simulink model "Tiltrotor_temp"  (R2017b)
settings: Solver=VariableStepAuto  StartTime=0.0  StopTime=60  RelTol=1e-3
PreLoadFcn:
  | parameter_Tiltrotor;
  | time;
InitFcn:
  | parameter_Tiltrotor;
  | time;
model workspace: external: MATLAB File E:\Matlab\CTRUAV_V1\parameter_Tiltrotor.m (data not in the file)
values from neighbouring files (symbols this model uses):
  Bm = 2    [parameter_Tiltrotor.m]
  Dm = 0.005    [parameter_Tiltrotor.m]
  Dphi = 0.01    [parameter_Tiltrotor.m]
  Dpsi = 0.01    [parameter_Tiltrotor.m]
  Ds = 15    [parameter_Tiltrotor.m]
  Dtheta = 0.01    [parameter_Tiltrotor.m]
  Dx = 0.04    [parameter_Tiltrotor.m]
  Dy = 0.04    [parameter_Tiltrotor.m]
  Dz = 0.08    [parameter_Tiltrotor.m]
  Im = 0.05    [parameter_Tiltrotor.m]
  Inheight = 0.1    [parameter_Tiltrotor.m]
  Is = 0    [parameter_Tiltrotor.m]
  Kdphi = 7    [parameter_Tiltrotor.m]
  Kdpsi = 4    [parameter_Tiltrotor.m]
  Kdtheta = 9    [parameter_Tiltrotor.m]
  Kdx = 5    [parameter_Tiltrotor.m]
  Kdy = 3    [parameter_Tiltrotor.m]
  Kdz = 6.5    [parameter_Tiltrotor.m]
  Kf = 0.04    [parameter_Tiltrotor.m]
  Kfv = 0.04    [parameter_Tiltrotor.m]
  Kphi = 7    [parameter_Tiltrotor.m]
  Kpsi = 4    [parameter_Tiltrotor.m]
  Ktheta = 9    [parameter_Tiltrotor.m]
  lb = 0.24    [parameter_Tiltrotor.m]
  lf = 0.078    [parameter_Tiltrotor.m]
  lh = 0.0142    [parameter_Tiltrotor.m]
  ls = 0.151    [parameter_Tiltrotor.m]
  m = 0.979    [parameter_Tiltrotor.m]
  Pm = 0.16    [parameter_Tiltrotor.m]
  Ps = 30    [parameter_Tiltrotor.m]
undefined symbols (not defined in the file or in its folder): sigbuilder_block, smiData, X, Y, Z
libraries: sm_lib x243, nesl_utility x48, simulink x8, fl_lib x4
(part 1 of 6)
settings Model: Creator=Lvzongyang  LastModifiedBy=lvzongyang

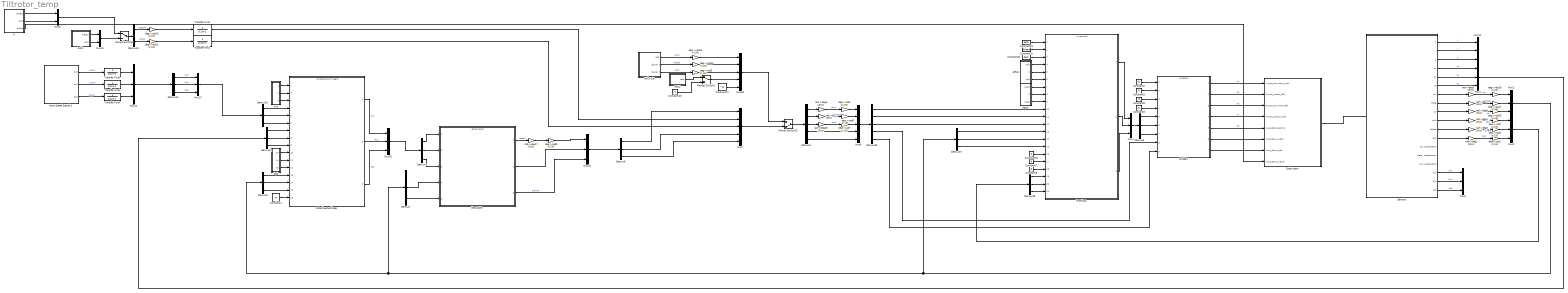
== system Tiltrotor_temp ==
  0 : Subsystem  Tag=STV Subsys  LoadFcn=sigbuilder_block('load');  StartFcn=sigbuilder_block('start');  StopFcn=sigbuilder_block('stop');  ClipboardFcn=sigbuilder_block('clipboard');  mask(Sigbuilder block){tuvar=[0:10]}
      mask help: Simulink:masks:SigbuilderBlock_MD
      mask init:
      | if ~strcmp(get_param(bdroot(gcbh),'SimulationStatus'),'stopped') tuvar = sigbuilder_block('maskInit'); end
      settings: CopyFcn=sigbuilder_block('copy');  DeleteFcn=sigbuilder_block('delete');  ModelCloseFcn=sigbuilder_block('modelClose');  PreSaveFcn=sigbuilder_block('preSave');  PauseFcn=sigbuilder_block('pause');  ContinueFcn=sigbuilder_block('continue');  NameChangeFcn=sigbuilder_block('namechange');  OpenFcn=sigbuilder_block('open',[1322.25 66 1162.5 420.75 ]);  CloseFcn=sigbuilder_block('close');
      mask Display: plot(0, 0, 100, 100,[2, 2, 32, 32, 2], [68, 8, 8, 68, 68],[32, 2], [38, 38], [32, 19, 2],[53, 60, 44], [32, 17, 17, 2],[16, 16, 31, 31]);txt = getActiveGroup(gcbh);text(2, 100, txt,'verticalAlignment', 'top');
  Constant1 : Constant  Value=m
  Constant{7,9..10,15} (4 alike) : Constant  Value=0
  Constant17 : Constant  Value=-11
  Constant19 : Constant  Value=Dphi
  Constant2 : Constant  Value=lb
  Constant20 : Constant  Value=Dtheta
  Constant21 : Constant  Value=Dpsi
  Constant3 : Constant  Value=lf
  Constant6 : Constant  Value=ls
  Constant8 : Constant  Value=lh
  Decoupler : ModelReference  ModelNameDialog=Decoupler0  ModelReferenceVersion=1.160  CopyOfModelProtected=on
  Demux10 : Demux  Outputs=2
  Demux{2..3,7..9,14,20..21,37,39} (10 alike) : Demux  Outputs=3
  Demux36 : Demux  Outputs=5
  Demux6 : Demux  Outputs=5
  Dp2 : Subsystem
  Input Speed Signals1 : Subsystem  Tag=STV Subsys  LoadFcn=sigbuilder_block('load');  StartFcn=sigbuilder_block('start');  StopFcn=sigbuilder_block('stop');  ClipboardFcn=sigbuilder_block('clipboard');  mask(Sigbuilder block){tuvar=[0:10]}
      mask help: Simulink:masks:SigbuilderBlock_MD
      mask init:
      | if ~strcmp(get_param(bdroot(gcbh),'SimulationStatus'),'stopped') tuvar = sigbuilder_block('maskInit'); end
      settings: CopyFcn=sigbuilder_block('copy');  DeleteFcn=sigbuilder_block('delete');  ModelCloseFcn=sigbuilder_block('modelClose');  PreSaveFcn=sigbuilder_block('preSave');  PauseFcn=sigbuilder_block('pause');  ContinueFcn=sigbuilder_block('continue');  NameChangeFcn=sigbuilder_block('namechange');  OpenFcn=sigbuilder_block('open',[57.75 0 966.75 517.5 ]);  CloseFcn=sigbuilder_block('close');
      mask Display: plot(0, 0, 100, 100,[2, 2, 32, 32, 2], [68, 8, 8, 68, 68],[32, 2], [38, 38], [32, 19, 2],[53, 60, 44], [32, 17, 17, 2],[16, 16, 31, 31]);txt = getActiveGroup(gcbh);text(2, 100, txt,'verticalAlignment', 'top');
  Kot : Subsystem
  MIXER1 : ModelReference  ModelNameDialog=MIXER10  ModelReferenceVersion=1.160  CopyOfModelProtected=on
  Manual Switch2 : ManualSwitch
  Manual Switch23 : ManualSwitch  CurrentSetting=0
  Manual Switch6 : ManualSwitch
  Mux{1..5,11..12,19,25,27} (10 alike) : Mux  Inputs=3
  Mux10 : Mux  Inputs=2
  Mux39 : Mux  Inputs=5
  Mux6 : Mux  Inputs=5
  Mux7 : Mux  Inputs=5
  Mux9 : Mux  Inputs=2
  "Outerloopnonlinear " : ModelReference  ModelNameDialog=Outerloopnonlinear0  ModelReferenceVersion=1.160  CopyOfModelProtected=on
  Roll1 : Subsystem  Tag=STV Subsys  LoadFcn=sigbuilder_block('load');  StartFcn=sigbuilder_block('start');  StopFcn=sigbuilder_block('stop');  ClipboardFcn=sigbuilder_block('clipboard');  mask(Sigbuilder block){tuvar=[0:10]}
      mask help: Simulink:masks:SigbuilderBlock_MD
      mask init:
      | if ~strcmp(get_param(bdroot(gcbh),'SimulationStatus'),'stopped') tuvar = sigbuilder_block('maskInit'); end
      settings: CopyFcn=sigbuilder_block('copy');  DeleteFcn=sigbuilder_block('delete');  ModelCloseFcn=sigbuilder_block('modelClose');  PreSaveFcn=sigbuilder_block('preSave');  PauseFcn=sigbuilder_block('pause');  ContinueFcn=sigbuilder_block('continue');  NameChangeFcn=sigbuilder_block('namechange');  OpenFcn=sigbuilder_block('open',[421.5 181.5 1012.5 423 ]);  CloseFcn=sigbuilder_block('close');
      mask Display: plot(0, 0, 100, 100,[2, 2, 32, 32, 2], [68, 8, 8, 68, 68],[32, 2], [38, 38], [32, 19, 2],[53, 60, 44], [32, 17, 17, 2],[16, 16, 31, 31]);txt = getActiveGroup(gcbh);text(2, 100, txt,'verticalAlignment', 'top');
  Roll3-10s : Subsystem  Tag=STV Subsys  LoadFcn=sigbuilder_block('load');  StartFcn=sigbuilder_block('start');  StopFcn=sigbuilder_block('stop');  ClipboardFcn=sigbuilder_block('clipboard');  mask(Sigbuilder block){tuvar=[0:10]}
      mask help: Simulink:masks:SigbuilderBlock_MD
      mask init:
      | if ~strcmp(get_param(bdroot(gcbh),'SimulationStatus'),'stopped') tuvar = sigbuilder_block('maskInit'); end
      settings: CopyFcn=sigbuilder_block('copy');  DeleteFcn=sigbuilder_block('delete');  ModelCloseFcn=sigbuilder_block('modelClose');  PreSaveFcn=sigbuilder_block('preSave');  PauseFcn=sigbuilder_block('pause');  ContinueFcn=sigbuilder_block('continue');  NameChangeFcn=sigbuilder_block('namechange');  OpenFcn=sigbuilder_block('open',[212.25 112.5 1012.5 505.5 ]);  CloseFcn=sigbuilder_block('close');
      mask Display: plot(0, 0, 100, 100,[2, 2, 32, 32, 2], [68, 8, 8, 68, 68],[32, 2], [38, 38], [32, 19, 2],[53, 60, 44], [32, 17, 17, 2],[16, 16, 31, 31]);txt = getActiveGroup(gcbh);text(2, 100, txt,'verticalAlignment', 'top');
  Roll4 : Subsystem  Tag=STV Subsys  LoadFcn=sigbuilder_block('load');  StartFcn=sigbuilder_block('start');  StopFcn=sigbuilder_block('stop');  ClipboardFcn=sigbuilder_block('clipboard');  mask(Sigbuilder block){tuvar=[0:10]}
      mask help: Simulink:masks:SigbuilderBlock_MD
      mask init:
      | if ~strcmp(get_param(bdroot(gcbh),'SimulationStatus'),'stopped') tuvar = sigbuilder_block('maskInit'); end
      settings: CopyFcn=sigbuilder_block('copy');  DeleteFcn=sigbuilder_block('delete');  ModelCloseFcn=sigbuilder_block('modelClose');  PreSaveFcn=sigbuilder_block('preSave');  PauseFcn=sigbuilder_block('pause');  ContinueFcn=sigbuilder_block('continue');  NameChangeFcn=sigbuilder_block('namechange');  OpenFcn=sigbuilder_block('open',[212.25 112.5 1012.5 505.5 ]);  CloseFcn=sigbuilder_block('close');
      mask Display: plot(0, 0, 100, 100,[2, 2, 32, 32, 2], [68, 8, 8, 68, 68],[32, 2], [38, 38], [32, 19, 2],[53, 60, 44], [32, 17, 17, 2],[16, 16, 31, 31]);txt = getActiveGroup(gcbh);text(2, 100, txt,'verticalAlignment', 'top');
  Sensors : Subsystem
  Subsystem : Subsystem
  Transfer Fcn{1,3,6,8..9} (5 alike) : TransferFcn  Denominator=[0.1 1]
  aeta1 : Subsystem
  aeta2 : Subsystem
  deg->rad{1..8,10..11,13..17} (15 alike) : Gain  Gain=pi/180
  innerloop : ModelReference  ModelNameDialog=innerloop0  ModelReferenceVersion=1.160  CopyOfModelProtected=on
  rad->deg{1..8,16..17} (10 alike) : Gain  Gain=180/pi
  wires:
  Sensors/12(dpsi) -> rad->deg2/1
  rad->deg5/1 -> deg->rad16/1  "phi"
  Sensors/11(dtheta) -> rad->deg3/1
  deg->rad2/1 -> Mux3/1
  deg->rad17/1 -> Mux2/2
  deg->rad15/1 -> Mux2/3
  Sensors/10(dphi) -> rad->deg1/1
  Sensors/9(psi) -> rad->deg6/1
  Sensors/8(theta) -> rad->deg7/1
  deg->rad16/1 -> Mux2/1
  deg->rad3/1 -> Mux3/2
  rad->deg1/1 -> deg->rad2/1  "dphi"
  rad->deg3/1 -> deg->rad3/1  "tdheta"
  rad->deg2/1 -> deg->rad1/1  "dpsi"
  Sensors/7(phi) -> rad->deg5/1
  deg->rad1/1 -> Mux3/3
  rad->deg6/1 -> deg->rad15/1  "psi"
  rad->deg7/1 -> deg->rad17/1  "theta"
  aeta2/2(Kdtheta) -> innerloop/8
  aeta2/1(Kdphi) -> innerloop/7
  Demux37/3 -> innerloop/15
  Roll3-10s/3(Signal 2) -> deg->rad5/1  "psid"
  Constant20/1 -> innerloop/2
  aeta2/3(Kdpsi) -> innerloop/9
  Constant7/1 -> innerloop/17
  Roll3-10s/1(test) -> deg->rad13/1  "phid"
  Constant15/1 -> innerloop/16
  Roll3-10s/2(Signal 1) -> deg->rad14/1  "thetad"
  Constant19/1 -> innerloop/1
  Demux39/3 -> innerloop/21
  aeta1/2(Ktheta) -> innerloop/5
  Demux36/2 -> innerloop/11
  Constant9/1 -> innerloop/18
  Demux37/2 -> innerloop/14
  Constant21/1 -> innerloop/3
  aeta1/1(Kphi) -> innerloop/4
  aeta1/3(Kpsi) -> innerloop/6
  Demux39/1 -> innerloop/19
  Demux39/2 -> innerloop/20
  Demux20/2 -> "Outerloopnonlinear "/5
  Demux14/2 -> Mux27/2  "dyd"
  "Outerloopnonlinear "/3 -> Mux25/3  "Fzd"
  deg->rad8/1 -> Mux19/1
  Demux14/1 -> Mux27/1  "dxd"
  Dp2/1(Dx) -> "Outerloopnonlinear "/10
  Mux27/1 -> Demux20/1
  Demux21/3 -> "Outerloopnonlinear "/9
  Demux2/1 -> Decoupler/1
  Dp2/3(Dz) -> "Outerloopnonlinear "/12
  Demux20/1 -> "Outerloopnonlinear "/4
  Demux21/2 -> "Outerloopnonlinear "/8
  Kot/1(Kdx) -> "Outerloopnonlinear "/1
  "Outerloopnonlinear "/1 -> Mux25/1  "Fxd"
  Demux14/3 -> Mux27/3  "dzd"
  Demux20/3 -> "Outerloopnonlinear "/6
  Decoupler/2 -> Mux19/2
  Mux19/1 -> Demux8/1
  Dp2/2(Dy) -> "Outerloopnonlinear "/11
  Demux2/3 -> Decoupler/3
  "Outerloopnonlinear "/2 -> Mux25/2  "Fyd"
  Demux2/2 -> Decoupler/2
  Decoupler/3 -> Mux19/3  "alphad"
  Decoupler/1 -> rad->deg17/1  "betad"
  Kot/2(Kdy) -> "Outerloopnonlinear "/2
  Demux21/1 -> "Outerloopnonlinear "/7
  Demux7/3 -> Decoupler/5
  Mux1/1 -> Demux21/1
  Demux7/2 -> Decoupler/4
  Mux3/1 -> Demux39/1
  Demux36/3 -> innerloop/12
  Mux39/1 -> Manual Switch23/1
  Constant8/1 -> MIXER1/4
  Constant6/1 -> MIXER1/3
  Constant3/1 -> MIXER1/2
  Constant2/1 -> MIXER1/1
  Demux36/4 -> MIXER1/8
  MIXER1/7 -> Subsystem/7(Input_Servo_left)
  MIXER1/4 -> Subsystem/4(4Input_uprotor_right)  "w4"
  MIXER1/3 -> Subsystem/3(3Input_downrotor_left)  "w3"
  MIXER1/2 -> Subsystem/2(2Input_uprotor_left)  "w2"
  MIXER1/1 -> Subsystem/1(1Input_downrotor_right)  "w1"
  MIXER1/5 -> Subsystem/5(Input_Rotor_behind)  "w5"
  MIXER1/6 -> Subsystem/6(Input_Servo_right)
  Demux3/2 -> MIXER1/6
  Demux3/1 -> MIXER1/5
  Demux3/3 -> MIXER1/7
  Mux4/1 -> Demux3/1
  innerloop/2 -> Mux4/2
  innerloop/1 -> Mux4/1
  innerloop/3 -> Mux4/3
  Demux36/1 -> innerloop/10
  Sensors/1(X) -> Mux11/1  "X"
  Sensors/2(Y) -> Mux11/2  "Y"
  Sensors/3(Z) -> Mux11/3  "Z"
  Sensors/4(dx) -> Mux1/1  "dx"
  Sensors/5(dy) -> Mux1/2  "dy"
  Sensors/6(dz) -> Mux1/3  "dz"
  Sensors/16(dxb) -> Mux5/1  "dxb"
  Sensors/17(dyb) -> Mux5/2  "dyb"
  Sensors/18(dzb) -> Mux5/3  "dzb"
  Demux36/5 -> MIXER1/9
  Manual Switch2/1 -> Mux39/4
  Constant17/1 -> Mux39/5
  Manual Switch23/1 -> Demux6/1
  Demux6/1 -> rad->deg4/1
  Demux6/2 -> rad->deg8/1
  Demux6/3 -> rad->deg16/1
  Demux6/4 -> Mux6/4
  Demux6/5 -> Mux6/5
  Mux6/1 -> Demux36/1
  deg->rad4/1 -> Mux6/1
  rad->deg4/1 -> deg->rad4/1  "phid"
  deg->rad6/1 -> Mux6/2
  rad->deg8/1 -> deg->rad6/1  "thetad"
  rad->deg16/1 -> deg->rad7/1  "psid"
  deg->rad7/1 -> Mux6/3
  Kot/3(Kdz) -> "Outerloopnonlinear "/3
  Constant1/1 -> "Outerloopnonlinear "/16
  Demux8/2 -> Mux7/4
  Demux8/3 -> Mux7/5
  Demux8/1 -> Mux7/1
  Mux7/1 -> Manual Switch23/2
  Roll1/1(thetad) -> Mux10/1
  Roll1/2(psid) -> Mux10/2
  Demux9/1 -> "Outerloopnonlinear "/13
  Demux9/2 -> "Outerloopnonlinear "/14
  Demux9/3 -> "Outerloopnonlinear "/15
  Mux2/1 -> Demux9/1, Demux7/1, Demux37/1
  rad->deg17/1 -> deg->rad8/1
  Constant10/1 -> Manual Switch2/2
  Roll4/1(test) -> Manual Switch2/1
  Mux25/1 -> Demux2/1
  deg->rad10/1 -> Transfer Fcn3/1
  deg->rad11/1 -> Transfer Fcn1/1
  Transfer Fcn3/1 -> Mux7/2
  Transfer Fcn1/1 -> Mux7/3
  0/1(thetad) -> Mux9/1
  0/2(psid) -> Mux9/2
  Mux10/1 -> Manual Switch6/2
  Mux9/1 -> Manual Switch6/1
  Manual Switch6/1 -> Demux10/1
  Demux10/1 -> deg->rad10/1  "thetad1"
  Demux10/2 -> deg->rad11/1  "psid1"
  deg->rad5/1 -> Mux39/3
  deg->rad13/1 -> Mux39/1
  deg->rad14/1 -> Mux39/2
  Mux12/1 -> Demux14/1
  Transfer Fcn9/1 -> Mux12/3
  Transfer Fcn6/1 -> Mux12/2
  Input Speed Signals1/2(dyd) -> Transfer Fcn6/1  "y_d_or"
  Transfer Fcn8/1 -> Mux12/1
  Input Speed Signals1/1(dxd) -> Transfer Fcn8/1  "x_d_or"
  Input Speed Signals1/3(dzd) -> Transfer Fcn9/1  "z_d_or"
  0/3(probe) -> Subsystem/8(Input_Servo_right1)
  Demux37/1 -> innerloop/13
  connections:
  Subsystem/RConn1 -- Sensors/LConn1

== system Tiltrotor_temp/0 ==
  Demux : Demux  Tag=STV Demux  Outputs=3
  FromWs : FromWorkspace  Tag=STV FromWs  VariableName=tuvar  SampleTime=0
      SigBuilderData=|
      | common.afterFinalStr = 'Extrapolate'
      | common.sampleTime = 0
      | dataSet.timeRange = [0 60]
      | dataSet.name = 'Group 1'
      | sbobj.Groups.Name = 'Group 1'
      | sbobj.Groups.Signals(1).Name = 'thetad'
      | sbobj.Groups.Signals(1).XData = [0 3 5 21 23 32 34 54 56 60]
      | sbobj.Groups.Signals(1).YData = [0 0 45 45 0.5 0.5 45 45 0 0]
      | sbobj.Groups.Signals(2).Name = 'psid'
      | sbobj.Groups.Signals(2).XData = [0 24 26 29 31 60]
      | sbobj.Groups.Signals(2).YData = [0 0 90 90 -1 -1]
      | sbobj.Groups.Signals(3).Name = 'probe'
      | sbobj.Groups.Signals(3).XData = [0 5.5 6 20 20.5 34.5 35 53 53.5 60]
      | sbobj.Groups.Signals(3).YData = [0 0 45 45 0 0 45 45 1 1]
      | sbobj.Groups.TimeRange = [0 60]
  thetad : Outport  Tag=STV Outport
  psid : Outport  Tag=STV Outport  Port=2
  probe : Outport  Tag=STV Outport  Port=3
  wires:
  FromWs/1 -> Demux/1
  Demux/1 -> thetad/1
  Demux/2 -> psid/1
  Demux/3 -> probe/1

== system Tiltrotor_temp/Dp2 ==
  Constant1 : Constant  Value=Dz
  Constant2 : Constant  Value=Dx
  Constant3 : Constant  Value=Dy
  Dx : Outport
  Dy : Outport  Port=2
  Dz : Outport  Port=3
  wires:
  Constant3/1 -> Dy/1
  Constant2/1 -> Dx/1
  Constant1/1 -> Dz/1

== system Tiltrotor_temp/Input Speed Signals1 ==
  Demux : Demux  Tag=STV Demux  Outputs=3
  FromWs : FromWorkspace  Tag=STV FromWs  VariableName=tuvar  SampleTime=0
      SigBuilderData=|
      | common.afterFinalStr = 'Extrapolate'
      | common.sampleTime = 0
      | dataSet.timeRange = [0 15]
      | dataSet.name = 'Group 1'
      | sbobj.Groups.Name = 'Group 1'
      | sbobj.Groups.Signals(1).Name = 'dxd'
      | sbobj.Groups.Signals(1).XData = [0 2 2 15]
      | sbobj.Groups.Signals(1).YData = [0 0 3 3]
      | sbobj.Groups.Signals(2).Name = 'dyd'
      | sbobj.Groups.Signals(2).XData = [0 5 5 15]
      | sbobj.Groups.Signals(2).YData = [0 0 2 2]
      | sbobj.Groups.Signals(3).Name = 'dzd'
      | sbobj.Groups.Signals(3).XData = [0 1 7 7 15]
      | sbobj.Groups.Signals(3).YData = [-1 -1 -1 -0.02 -0.02]
      | sbobj.Groups.TimeRange = [0 15]
  dxd : Outport  Tag=STV Outport
  dyd : Outport  Tag=STV Outport  Port=2
  dzd : Outport  Tag=STV Outport  Port=3
  wires:
  FromWs/1 -> Demux/1
  Demux/1 -> dxd/1
  Demux/2 -> dyd/1
  Demux/3 -> dzd/1

== system Tiltrotor_temp/Kot ==
  Constant1 : Constant  Value=Kdz
  Constant2 : Constant  Value=Kdx
  Constant3 : Constant  Value=Kdy
  Kdx : Outport
  Kdy : Outport  Port=2
  Kdz : Outport  Port=3
  wires:
  Constant3/1 -> Kdy/1
  Constant2/1 -> Kdx/1
  Constant1/1 -> Kdz/1

== system Tiltrotor_temp/Roll1 ==
  Demux : Demux  Tag=STV Demux  Outputs=2
  FromWs : FromWorkspace  Tag=STV FromWs  VariableName=tuvar  SampleTime=0
      SigBuilderData=|
      | common.afterFinalStr = 'Extrapolate'
      | common.sampleTime = 0
      | dataSet.timeRange = [0 15]
      | dataSet.name = 'Group 1'
      | sbobj.Groups.Name = 'Group 1'
      | sbobj.Groups.Signals(1).Name = 'thetad'
      | sbobj.Groups.Signals(1).XData = [0 12 12 15]
      | sbobj.Groups.Signals(1).YData = [0 0 30 30]
      | sbobj.Groups.Signals(2).Name = 'psid'
      | sbobj.Groups.Signals(2).XData = [0 9 9 15]
      | sbobj.Groups.Signals(2).YData = [0 0 20 20]
      | sbobj.Groups.TimeRange = [0 15]
  thetad : Outport  Tag=STV Outport
  psid : Outport  Tag=STV Outport  Port=2
  wires:
  FromWs/1 -> Demux/1
  Demux/1 -> thetad/1
  Demux/2 -> psid/1

== system Tiltrotor_temp/Roll3-10s ==
  Demux : Demux  Tag=STV Demux  Outputs=3
  FromWs : FromWorkspace  Tag=STV FromWs  VariableName=tuvar  SampleTime=0
      SigBuilderData=|
      | common.afterFinalStr = 'Extrapolate'
      | common.sampleTime = 0
      | dataSet.timeRange = [0 10]
      | dataSet.name = 'Group 1'
      | sbobj.Groups.Name = 'Group 1'
      | sbobj.Groups.Signals(1).Name = 'test'
      | sbobj.Groups.Signals(1).XData = [0 1 1 10]
      | sbobj.Groups.Signals(1).YData = [0 0 20 20]
      | sbobj.Groups.Signals(2).Name = 'Signal 1'
      | sbobj.Groups.Signals(2).XData = [0 3 3 10]
      | sbobj.Groups.Signals(2).YData = [0 0 15 15]
      | sbobj.Groups.Signals(3).Name = 'Signal 2'
      | sbobj.Groups.Signals(3).XData = [0 5 5 10]
      | sbobj.Groups.Signals(3).YData = [0 0 30 30]
  test : Outport  Tag=STV Outport
  Signal 1 : Outport  Tag=STV Outport  Port=2
  Signal 2 : Outport  Tag=STV Outport  Port=3
  wires:
  FromWs/1 -> Demux/1
  Demux/1 -> test/1
  Demux/2 -> Signal 1/1
  Demux/3 -> Signal 2/1

== system Tiltrotor_temp/Roll4 ==
  Demux : Demux  Tag=STV Demux  Outputs=1
  FromWs : FromWorkspace  Tag=STV FromWs  VariableName=tuvar  SampleTime=0
      SigBuilderData=|
      | common.afterFinalStr = 'Extrapolate'
      | common.sampleTime = 0
      | dataSet.timeRange = [0 10]
      | dataSet.name = 'Group 1'
      | sbobj.Groups.Name = 'Group 1'
      | sbobj.Groups.Signals.Name = 'test'
      | sbobj.Groups.Signals.XData = [0 7 7 10]
      | sbobj.Groups.Signals.YData = [0 0 0.2 0.2]
  test : Outport  Tag=STV Outport
  wires:
  FromWs/1 -> Demux/1
  Demux/1 -> test/1

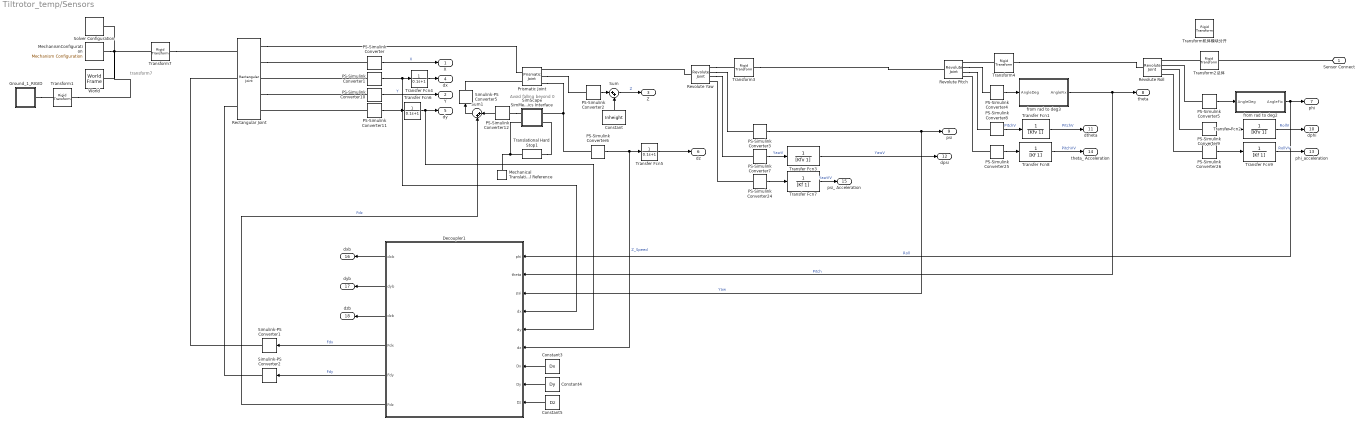
== system Tiltrotor_temp/Sensors ==
  note: Avoid falling beyond 0
  note: transform7
  Constant : Constant  Value=Inheight
  Constant3 : Constant  Value=Dx
  Constant4 : Constant  Value=Dy
  Constant5 : Constant  Value=Dz
  Decoupler1 : MATLAB Function  TreatAsAtomicUnit=on
  Ground_1_RIGID : Subsystem
  Mechanical Translational Reference : fl_lib/Mechanical/Translational Elements/Mechanical Translational Reference
  MechanismConfiguration : sm_lib/Utilities/Mechanism Configuration  UniformGravity=Constant  GravityVector=[0 0 -9.80665]  GravityUnits=m/s^2  LinearizationDelta=0.001
  PS-Simulink Converter : nesl_utility/PS-Simulink Converter  PhysicalDomain=network_engine_domain  SubClassName=ps_output  LeftPortType=input  RightPortType=output  PseudoPeriodic=off  Frequencies=[]  Unit=m  AffineConversion=off
  PS-Simulink Converter1 : nesl_utility/PS-Simulink Converter  PhysicalDomain=network_engine_domain  SubClassName=ps_output  LeftPortType=input  RightPortType=output  PseudoPeriodic=off  Frequencies=[]  Unit=m/s  AffineConversion=off
  PS-Simulink Converter10 : nesl_utility/PS-Simulink Converter  PhysicalDomain=network_engine_domain  SubClassName=ps_output  LeftPortType=input  RightPortType=output  PseudoPeriodic=off  Frequencies=[]  Unit=m  AffineConversion=off
  PS-Simulink Converter11 : nesl_utility/PS-Simulink Converter  PhysicalDomain=network_engine_domain  SubClassName=ps_output  LeftPortType=input  RightPortType=output  PseudoPeriodic=off  Frequencies=[]  Unit=m/s  AffineConversion=off
  PS-Simulink Converter12 : nesl_utility/PS-Simulink Converter  PhysicalDomain=network_engine_domain  SubClassName=ps_output  LeftPortType=input  RightPortType=output  PseudoPeriodic=off  Frequencies=[]  Unit=N  AffineConversion=off
  PS-Simulink Converter2 : nesl_utility/PS-Simulink Converter  PhysicalDomain=network_engine_domain  SubClassName=ps_output  LeftPortType=input  RightPortType=output  PseudoPeriodic=off  Frequencies=[]  Unit=m  AffineConversion=off
  PS-Simulink Converter24 : nesl_utility/PS-Simulink Converter  PhysicalDomain=network_engine_domain  SubClassName=ps_output  LeftPortType=input  RightPortType=output  PseudoPeriodic=off  Frequencies=[]  Unit=rad/s^2  AffineConversion=off
  PS-Simulink Converter25 : nesl_utility/PS-Simulink Converter  PhysicalDomain=network_engine_domain  SubClassName=ps_output  LeftPortType=input  RightPortType=output  PseudoPeriodic=off  Frequencies=[]  Unit=rad/s^2  AffineConversion=off
  PS-Simulink Converter26 : nesl_utility/PS-Simulink Converter  PhysicalDomain=network_engine_domain  SubClassName=ps_output  LeftPortType=input  RightPortType=output  PseudoPeriodic=off  Frequencies=[]  Unit=rad/s^2  AffineConversion=off
  PS-Simulink Converter3 : nesl_utility/PS-Simulink Converter  PhysicalDomain=network_engine_domain  SubClassName=ps_output  LeftPortType=input  RightPortType=output  PseudoPeriodic=off  Frequencies=[]  Unit=rad  AffineConversion=off
  PS-Simulink Converter4 : nesl_utility/PS-Simulink Converter  PhysicalDomain=network_engine_domain  SubClassName=ps_output  LeftPortType=input  RightPortType=output  PseudoPeriodic=off  Frequencies=[]  Unit=rad  AffineConversion=off
  PS-Simulink Converter5 : nesl_utility/PS-Simulink Converter  PhysicalDomain=network_engine_domain  SubClassName=ps_output  LeftPortType=input  RightPortType=output  PseudoPeriodic=off  Frequencies=[]  Unit=rad  AffineConversion=off
  PS-Simulink Converter6 : nesl_utility/PS-Simulink Converter  PhysicalDomain=network_engine_domain  SubClassName=ps_output  LeftPortType=input  RightPortType=output  PseudoPeriodic=off  Frequencies=[]  Unit=m/s  AffineConversion=off
  PS-Simulink Converter7 : nesl_utility/PS-Simulink Converter  PhysicalDomain=network_engine_domain  SubClassName=ps_output  LeftPortType=input  RightPortType=output  PseudoPeriodic=off  Frequencies=[]  Unit=rad/s  AffineConversion=off
  PS-Simulink Converter8 : nesl_utility/PS-Simulink Converter  PhysicalDomain=network_engine_domain  SubClassName=ps_output  LeftPortType=input  RightPortType=output  PseudoPeriodic=off  Frequencies=[]  Unit=rad/s  AffineConversion=off
  PS-Simulink Converter9 : nesl_utility/PS-Simulink Converter  PhysicalDomain=network_engine_domain  SubClassName=ps_output  LeftPortType=input  RightPortType=output  PseudoPeriodic=off  Frequencies=[]  Unit=rad/s  AffineConversion=off
  Prismatic Joint : sm_lib/Joints/Prismatic Joint  SenseConstraintForce=off  SenseConstraintForceX=off  SenseConstraintForceY=off  SenseConstraintForceZ=off  SenseConstraintTorque=off  SenseConstraintTorqueX=off  SenseConstraintTorqueY=off  SenseConstraintTorqueZ=off  SenseTotalForce=off  SenseTotalForceX=off  SenseTotalForceY=off  SenseTotalForceZ=off  SenseTotalTorque=off  SenseTotalTorqueX=off  SenseTotalTorqueY=off  SenseTotalTorqueZ=off  CompositeWrenchDir=FollowerOnBase  CompositeWrenchFrame=BaseFrame  EquilibriumPosition=0  EquilibriumPositionUnits=m  SpringStiffness=0  SpringStiffnessUnits=N/m  DampingCoefficient=0  DampingCoefficientUnits=N/(m/s)  TorqueActuationMode=InputTorque  MotionActuationMode=ComputedMotion  SensePosition=on  SenseVelocity=on  SenseAcceleration=off  SenseTorqueForce=off  PositionTargetSpecify=off  PositionTargetPriority=High  PositionTargetValue=0  PositionTargetValueUnits=m  VelocityTargetSpecify=off  VelocityTargetPriority=High  VelocityTargetValue=0  VelocityTargetValueUnits=m/s
  Rectangular Joint : sm_lib/Joints/Rectangular Joint  SenseConstraintForce=off  SenseConstraintForceX=off  SenseConstraintForceY=off  SenseConstraintForceZ=off  SenseConstraintTorque=off  SenseConstraintTorqueX=off  SenseConstraintTorqueY=off  SenseConstraintTorqueZ=off  SenseTotalForce=off  SenseTotalForceX=off  SenseTotalForceY=off  SenseTotalForceZ=off  SenseTotalTorque=off  SenseTotalTorqueX=off  SenseTotalTorqueY=off  SenseTotalTorqueZ=off  CompositeWrenchDir=FollowerOnBase  CompositeWrenchFrame=BaseFrame  PxEquilibriumPosition=0  PxEquilibriumPositionUnits=m  PxSpringStiffness=0  PxSpringStiffnessUnits=N/m  PxDampingCoefficient=0  PxDampingCoefficientUnits=N/(m/s)  PxTorqueActuationMode=InputTorque  PxMotionActuationMode=ComputedMotion  PxSensePosition=on  PxSenseVelocity=on  PxSenseAcceleration=off  PxSenseTorqueForce=off  PxPositionTargetSpecify=off  PxPositionTargetPriority=High  PxPositionTargetValue=0  PxPositionTargetValueUnits=m  PxVelocityTargetSpecify=off  PxVelocityTargetPriority=High  PxVelocityTargetValue=0  PxVelocityTargetValueUnits=m/s  PyEquilibriumPosition=0  PyEquilibriumPositionUnits=m  PySpringStiffness=0  PySpringStiffnessUnits=N/m  PyDampingCoefficient=0  PyDampingCoefficientUnits=N/(m/s)  PyTorqueActuationMode=InputTorque  PyMotionActuationMode=ComputedMotion  PySensePosition=on  PySenseVelocity=on  PySenseAcceleration=off  PySenseTorqueForce=off  PyPositionTargetSpecify=off  PyPositionTargetPriority=High  PyPositionTargetValue=0  PyPositionTargetValueUnits=m  PyVelocityTargetSpecify=off  PyVelocityTargetPriority=High  PyVelocityTargetValue=0  PyVelocityTargetValueUnits=m/s
      settings: SourceProductName=Simscape Multibody
  Revolute Pitch : sm_lib/Joints/Revolute Joint  SenseConstraintForce=off  SenseConstraintForceX=off  SenseConstraintForceY=off  SenseConstraintForceZ=off  SenseConstraintTorque=off  SenseConstraintTorqueX=off  SenseConstraintTorqueY=off  SenseConstraintTorqueZ=off  SenseTotalForce=off  SenseTotalForceX=off  SenseTotalForceY=off  SenseTotalForceZ=off  SenseTotalTorque=off  SenseTotalTorqueX=off  SenseTotalTorqueY=off  SenseTotalTorqueZ=off  CompositeWrenchDir=FollowerOnBase  CompositeWrenchFrame=BaseFrame  EquilibriumPosition=0  EquilibriumPositionUnits=deg  SpringStiffness=0  SpringStiffnessUnits=N*m/deg  DampingCoefficient=Dtheta  DampingCoefficientUnits=N*m/(rad/s)  TorqueActuationMode=NoTorque  MotionActuationMode=ComputedMotion  SensePosition=on  SenseVelocity=on  SenseAcceleration=on  SenseTorqueForce=off  PositionTargetSpecify=off  PositionTargetPriority=High  PositionTargetValue=0  PositionTargetValueUnits=deg  VelocityTargetSpecify=off  VelocityTargetPriority=High  VelocityTargetValue=0  VelocityTargetValueUnits=deg/s
  Revolute Roll : sm_lib/Joints/Revolute Joint  SenseConstraintForce=off  SenseConstraintForceX=off  SenseConstraintForceY=off  SenseConstraintForceZ=off  SenseConstraintTorque=off  SenseConstraintTorqueX=off  SenseConstraintTorqueY=off  SenseConstraintTorqueZ=off  SenseTotalForce=off  SenseTotalForceX=off  SenseTotalForceY=off  SenseTotalForceZ=off  SenseTotalTorque=off  SenseTotalTorqueX=off  SenseTotalTorqueY=off  SenseTotalTorqueZ=off  CompositeWrenchDir=FollowerOnBase  CompositeWrenchFrame=BaseFrame  EquilibriumPosition=0  EquilibriumPositionUnits=deg  SpringStiffness=0  SpringStiffnessUnits=N*m/deg  DampingCoefficient=Dphi  DampingCoefficientUnits=N*m/(rad/s)  TorqueActuationMode=NoTorque  MotionActuationMode=ComputedMotion  SensePosition=on  SenseVelocity=on  SenseAcceleration=on  SenseTorqueForce=off  PositionTargetSpecify=off  PositionTargetPriority=High  PositionTargetValue=0  PositionTargetValueUnits=deg  VelocityTargetSpecify=off  VelocityTargetPriority=High  VelocityTargetValue=0  VelocityTargetValueUnits=deg/s
  Revolute Yaw : sm_lib/Joints/Revolute Joint  SenseConstraintForce=off  SenseConstraintForceX=off  SenseConstraintForceY=off  SenseConstraintForceZ=off  SenseConstraintTorque=off  SenseConstraintTorqueX=off  SenseConstraintTorqueY=off  SenseConstraintTorqueZ=off  SenseTotalForce=off  SenseTotalForceX=off  SenseTotalForceY=off  SenseTotalForceZ=off  SenseTotalTorque=off  SenseTotalTorqueX=off  SenseTotalTorqueY=off  SenseTotalTorqueZ=off  CompositeWrenchDir=FollowerOnBase  CompositeWrenchFrame=BaseFrame  EquilibriumPosition=0  EquilibriumPositionUnits=deg  SpringStiffness=0  SpringStiffnessUnits=N*m/deg  DampingCoefficient=Dpsi  DampingCoefficientUnits=N*m/(rad/s)  TorqueActuationMode=NoTorque  MotionActuationMode=ComputedMotion  SensePosition=on  SenseVelocity=on  SenseAcceleration=on  SenseTorqueForce=off  PositionTargetSpecify=off  PositionTargetPriority=High  PositionTargetValue=90  PositionTargetValueUnits=deg  VelocityTargetSpecify=off  VelocityTargetPriority=High  VelocityTargetValue=0  VelocityTargetValueUnits=deg/s
  SimScape SimMechanics Interface : Subsystem
  Simulink-PS Converter1 : nesl_utility/Simulink-PS Converter  PhysicalDomain=network_engine_domain  SubClassName=ps_input  LeftPortType=input  RightPortType=output  PseudoPeriodic=off  Frequencies=[]  NoiseDistribution=none  NoiseParameters=[]  Unit=N  AffineConversion=off  FilteringAndDerivatives=provide  SimscapeFilterOrder=1  InputFilterTimeConstant=0.001  UdotUserProvided=0
  Simulink-PS Converter2 : nesl_utility/Simulink-PS Converter  PhysicalDomain=network_engine_domain  SubClassName=ps_input  LeftPortType=input  RightPortType=output  PseudoPeriodic=off  Frequencies=[]  NoiseDistribution=none  NoiseParameters=[]  Unit=N  AffineConversion=off  FilteringAndDerivatives=provide  SimscapeFilterOrder=1  InputFilterTimeConstant=0.001  UdotUserProvided=0
  Simulink-PS Converter5 : nesl_utility/Simulink-PS Converter  PhysicalDomain=network_engine_domain  SubClassName=ps_input  LeftPortType=input  RightPortType=output  PseudoPeriodic=off  Frequencies=[]  NoiseDistribution=none  NoiseParameters=[]  Unit=N  AffineConversion=off  FilteringAndDerivatives=provide  SimscapeFilterOrder=1  InputFilterTimeConstant=0.001  UdotUserProvided=0
  Solver Configuration : nesl_utility/Solver Configuration  PhysicalDomain=network_engine_domain  SubClassName=solver  LeftPortType=input  RightPortType=generic  Accelerate=off  Tones=[]  Harmonics=[]  SimulateNoise=off  Profile=off  UseLocalSampling=off  EnableSwitchedLinearOptims=on  FrequencyDomain=off  UseCCode=off  RelTol=0.001  AbsTol=1e-06  MinStep=1e-09  ToWorkspace=off  RevertToSquareIcSolve=off  NumHomotopyIterations=100  PhasorMode=off  PhasorModeNumHarmonics=1  DoDC=on  ResidualTolerance=1e-09  UseLocalSolver=off  LocalSolverChoice=NE_BACKWARD_EULER_ADVANCER  LocalSolverSampleTime=0.001  DoFixedCost=off  MaxNonlinIter=3  MaxModeIter=2  LinearAlgebra=Sparse  DelaysMemoryBudget=1024  AutomaticFiltering=on  FilteringTimeConstant=0.001
  Sum : Sum  Inputs=|++
  Sum1 : Sum  Inputs=|++
  Transfer Fcn1 : TransferFcn  Denominator=[Kfv 1]
  Transfer Fcn2 : TransferFcn  Denominator=[Kfv 1]
  Transfer Fcn3 : TransferFcn  Denominator=[Kfv 1]
  Transfer Fcn4 : TransferFcn  Denominator=[0.1 1]
  Transfer Fcn5 : TransferFcn  Denominator=[0.1 1]
  Transfer Fcn6 : TransferFcn  Denominator=[0.1 1]
  Transfer Fcn7 : TransferFcn  Denominator=[Kf 1]
  Transfer Fcn8 : TransferFcn  Denominator=[Kf 1]
  Transfer Fcn9 : TransferFcn  Denominator=[Kf 1]
  Transform1 : sm_lib/Frames and Transforms/Rigid Transform  TranslationMethod=Cartesian  TranslationStandardOffset=0  TranslationLengthUnit=m  TranslationStandardAxis=+Z  TranslationCartesianOffset=[-4 4 -0.2]  TranslationROffset=0  TranslationROffsetUnits=m  TranslationZOffset=0  TranslationZOffsetUnits=m  TranslationThetaOffset=0  TranslationThetaOffsetUnits=deg  RotationMethod=None  RotationAngleUnits=deg  RotationStandardAxis=+Z  RotationAngle=0  RotationArbitraryAxis=[0 0 1]  FollAlignAxisA=+X  BaseAlignAxisA=+Y  FollAlignAxisB=+Y  BaseAlignAxisB=+Z  RotationSequenceAxes=FollowerAxes  RotationSequence=XYX  RotationSequenceAngles=[0 0 0]  RotationSequenceAnglesUnits=deg  RotationMatrix=[1 0 0; 0 1 0; 0 0 1]
  Transform2总体 : sm_lib/Frames and Transforms/Rigid Transform  TranslationMethod=Cartesian  TranslationStandardOffset=0  TranslationLengthUnit=m  TranslationStandardAxis=+Z  TranslationCartesianOffset=[0 -0.0143 -0.056]  TranslationROffset=0  TranslationROffsetUnits=m  TranslationZOffset=0  TranslationZOffsetUnits=m  TranslationThetaOffset=0  TranslationThetaOffsetUnits=deg  RotationMethod=StandardAxis  RotationAngleUnits=deg  RotationStandardAxis=+X  RotationAngle=90  RotationArbitraryAxis=[1 0 0]  FollAlignAxisA=+X  BaseAlignAxisA=+Y  FollAlignAxisB=+Y  BaseAlignAxisB=+Z  RotationSequenceAxes=FollowerAxes  RotationSequence=XYX  RotationSequenceAngles=[0 0 0]  RotationSequenceAnglesUnits=deg  RotationMatrix=[1 0 0; 0 1 0; 0 0 1]
  Transform3 : sm_lib/Frames and Transforms/Rigid Transform  TranslationMethod=Cartesian  TranslationStandardOffset=0  TranslationLengthUnit=m  TranslationStandardAxis=+Z  TranslationCartesianOffset=[0 0 0]  TranslationROffset=0  TranslationROffsetUnits=m  TranslationZOffset=0  TranslationZOffsetUnits=m  TranslationThetaOffset=0  TranslationThetaOffsetUnits=deg  RotationMethod=StandardAxis  RotationAngleUnits=deg  RotationStandardAxis=+X  RotationAngle=-90  RotationArbitraryAxis=[1 0 0]  FollAlignAxisA=+X  BaseAlignAxisA=+Y  FollAlignAxisB=+Y  BaseAlignAxisB=+Z  RotationSequenceAxes=FollowerAxes  RotationSequence=XYX  RotationSequenceAngles=[0 0 0]  RotationSequenceAnglesUnits=deg  RotationMatrix=[1 0 0; 0 1 0; 0 0 1]
  Transform4 : sm_lib/Frames and Transforms/Rigid Transform  TranslationMethod=Cartesian  TranslationStandardOffset=0  TranslationLengthUnit=m  TranslationStandardAxis=+Z  TranslationCartesianOffset=[0 0 0]  TranslationROffset=0  TranslationROffsetUnits=m  TranslationZOffset=0  TranslationZOffsetUnits=m  TranslationThetaOffset=0  TranslationThetaOffsetUnits=deg  RotationMethod=StandardAxis  RotationAngleUnits=deg  RotationStandardAxis=+Y  RotationAngle=90  RotationArbitraryAxis=[1 0 0]  FollAlignAxisA=+X  BaseAlignAxisA=+Y  FollAlignAxisB=+Y  BaseAlignAxisB=+Z  RotationSequenceAxes=FollowerAxes  RotationSequence=XYX  RotationSequenceAngles=[0 0 0]  RotationSequenceAnglesUnits=deg  RotationMatrix=[1 0 0; 0 1 0; 0 0 1]
  Transform7 : sm_lib/Frames and Transforms/Rigid Transform  TranslationMethod=Cartesian  TranslationStandardOffset=0  TranslationLengthUnit=mm  TranslationStandardAxis=+Z  TranslationCartesianOffset=[0 0 0]  TranslationROffset=0  TranslationROffsetUnits=m  TranslationZOffset=0  TranslationZOffsetUnits=m  TranslationThetaOffset=0  TranslationThetaOffsetUnits=deg  RotationMethod=ArbitraryAxis  RotationAngleUnits=rad  RotationStandardAxis=+Z  RotationAngle=pi  RotationArbitraryAxis=[1 0 0]  FollAlignAxisA=+X  BaseAlignAxisA=+Y  FollAlignAxisB=+Y  BaseAlignAxisB=+Z  RotationSequenceAxes=FollowerAxes  RotationSequence=XYX  RotationSequenceAngles=[0 0 0]  RotationSequenceAnglesUnits=deg  RotationMatrix=[1 0 0; 0 1 0; 0 0 1]
  Transform机体模块分开 : sm_lib/Frames and Transforms/Rigid Transform  TranslationMethod=Cartesian  TranslationStandardOffset=0  TranslationLengthUnit=m  TranslationStandardAxis=+Z  TranslationCartesianOffset=[0 0 -0.032]  TranslationROffset=0  TranslationROffsetUnits=m  TranslationZOffset=0  TranslationZOffsetUnits=m  TranslationThetaOffset=0  TranslationThetaOffsetUnits=deg  RotationMethod=StandardAxis  RotationAngleUnits=deg  RotationStandardAxis=+X  RotationAngle=90  RotationArbitraryAxis=[1 0 0]  FollAlignAxisA=+X  BaseAlignAxisA=+Y  FollAlignAxisB=+Y  BaseAlignAxisB=+Z  RotationSequenceAxes=FollowerAxes  RotationSequence=XYX  RotationSequenceAngles=[0 0 0]  RotationSequenceAnglesUnits=deg  RotationMatrix=[1 0 0; 0 1 0; 0 0 1]
  Translational Hard Stop1 : fl_lib/Mechanical/Translational Elements/Translational Hard Stop  upper_bnd=1000 m  lower_bnd=-Inheight m  stiff_up=1e3 N/m  stiff_low=1e3 N/m  D_up=150 N/(m/s)  D_low=150 N/(m/s)  model=3  transition=0.1 mm  v_specify=off  v_priority=None  v=0 m/s  v_nominal_specify=off  v_nominal_unit=m/s  v_nominal_value=1  f_specify=off  f_priority=None  f=0 N  f_nominal_specify=off  f_nominal_unit=N  f_nominal_value=1  x_specify=on  x_priority=High  x=0 m  x_nominal_specify=off  x_nominal_unit=m  x_nominal_value=1
  World : sm_lib/Frames and Transforms/World Frame
  from rad to deg2 : MATLAB Function  TreatAsAtomicUnit=on
  from rad to deg3 : MATLAB Function  TreatAsAtomicUnit=on
  Sensor Connect : PMIOPort  Port=1  Side=Left
  X : Outport
  Y : Outport  Port=2
  Z : Outport  Port=3
  dx : Outport  Port=4
  dy : Outport  Port=5
  dz : Outport  Port=6
  phi : Outport  Port=7
  theta : Outport  Port=8
  psi : Outport  Port=9
  dphi : Outport  Port=10
  dtheta : Outport  Port=11
  dpsi : Outport  Port=12
  phi_acceleration : Outport  Port=13
  theta_ Acceleration : Outport  Port=14
  psi_ Acceleration : Outport  Port=15
  dxb : Outport  Port=16
  dyb : Outport  Port=17
  dzb : Outport  Port=18
  wires:
  PS-Simulink Converter26/1 -> Transfer Fcn9/1
  Transfer Fcn8/1 -> theta_ Acceleration/1  "PitchVV"
  from rad to deg3/1(AngleFix) -> Decoupler1/2(theta), theta/1  "Pitch"
  PS-Simulink Converter24/1 -> Transfer Fcn7/1
  PS-Simulink Converter25/1 -> Transfer Fcn8/1
  from rad to deg2/1(AngleFix) -> phi/1, Decoupler1/1(phi)  "Roll"
  PS-Simulink Converter8/1 -> Transfer Fcn1/1  "PitchV"
  PS-Simulink Converter9/1 -> Transfer Fcn2/1
  Transfer Fcn7/1 -> psi_ Acceleration/1  "YawVV"
  PS-Simulink Converter7/1 -> Transfer Fcn3/1  "YawV"
  Transfer Fcn9/1 -> phi_acceleration/1  "RollVV"
  Transfer Fcn1/1 -> dtheta/1  "PitchV"
  PS-Simulink Converter3/1 -> psi/1, Decoupler1/3(psi)  "Yaw"
  Transfer Fcn3/1 -> dpsi/1  "YawV"
  PS-Simulink Converter6/1 -> Decoupler1/6(dz), Transfer Fcn5/1  "Z_Speed"
  PS-Simulink Converter11/1 -> Transfer Fcn6/1
  Constant/1 -> Sum/2
  PS-Simulink Converter4/1 -> from rad to deg3/1(AngleDeg)
  PS-Simulink Converter/1 -> X/1  "X"
  PS-Simulink Converter2/1 -> Sum/1
  PS-Simulink Converter10/1 -> Y/1  "Y"
  Transfer Fcn2/1 -> dphi/1  "RollV"
  Sum/1 -> Z/1  "Z"
  PS-Simulink Converter5/1 -> from rad to deg2/1(AngleDeg)
  Constant4/1 -> Decoupler1/8(Dy)
  Constant5/1 -> Decoupler1/9(Dz)
  Constant3/1 -> Decoupler1/7(Dx)
  Decoupler1/4(Fdx) -> Simulink-PS Converter1/1  "Fdx"
  Decoupler1/6(Fdz) -> Sum1/2  "Fdz"
  Decoupler1/5(Fdy) -> Simulink-PS Converter2/1  "Fdy"
  PS-Simulink Converter12/1 -> Sum1/1
  Sum1/1 -> Simulink-PS Converter5/1
  Decoupler1/1(dxb) -> dxb/1
  Decoupler1/2(dyb) -> dyb/1
  Decoupler1/3(dzb) -> dzb/1
  PS-Simulink Converter1/1 -> Transfer Fcn4/1, Decoupler1/4(dx)
  Transfer Fcn5/1 -> dz/1
  Transfer Fcn4/1 -> dx/1
  Transfer Fcn6/1 -> dy/1, Decoupler1/5(dy)
  connections:
  Mechanical Translational Reference/LConn1 -- Translational Hard Stop1/LConn1 -- SimScape SimMechanics Interface/LConn2
  Transform7/RConn1 -- Rectangular Joint/LConn1
  PS-Simulink Converter6/LConn1 -- SimScape SimMechanics Interface/RConn1 -- Prismatic Joint/RConn3
  PS-Simulink Converter1/LConn1 -- Rectangular Joint/RConn3
  PS-Simulink Converter25/LConn1 -- Revolute Pitch/RConn4
  Revolute Yaw/RConn1 -- Transform3/LConn1
  PS-Simulink Converter11/LConn1 -- Rectangular Joint/RConn5
  Prismatic Joint/LConn2 -- Simulink-PS Converter5/RConn1
  Rectangular Joint/RConn1 -- Prismatic Joint/LConn1
  PS-Simulink Converter26/LConn1 -- Revolute Roll/RConn4
  PS-Simulink Converter24/LConn1 -- Revolute Yaw/RConn4
  Rectangular Joint/RConn4 -- PS-Simulink Converter10/LConn1
  Rectangular Joint/RConn2 -- PS-Simulink Converter/LConn1
  Ground_1_RIGID/LConn1 -- Transform1/RConn1
  Revolute Pitch/RConn3 -- PS-Simulink Converter8/LConn1
  Revolute Yaw/RConn3 -- PS-Simulink Converter7/LConn1
  Revolute Yaw/RConn2 -- PS-Simulink Converter3/LConn1
  Revolute Pitch/RConn2 -- PS-Simulink Converter4/LConn1
  Prismatic Joint/RConn2 -- PS-Simulink Converter2/LConn1
  Revolute Yaw/LConn1 -- Prismatic Joint/RConn1
  PS-Simulink Converter5/LConn1 -- Revolute Roll/RConn2
  Transform4/LConn1 -- Revolute Pitch/RConn1
  Translational Hard Stop1/RConn1 -- SimScape SimMechanics Interface/RConn2
  Transform4/RConn1 -- Revolute Roll/LConn1
  Transform3/RConn1 -- Revolute Pitch/LConn1
  PS-Simulink Converter9/LConn1 -- Revolute Roll/RConn3
  MechanismConfiguration/RConn1 -- Transform7/LConn1 -- Transform1/LConn1 -- World/RConn1 -- Solver Configuration/RConn1
  Transform2总体/LConn1 -- Revolute Roll/RConn1
  Sensor Connect/RConn1 -- Transform2总体/RConn1
  Simulink-PS Converter1/RConn1 -- Rectangular Joint/LConn2
  Simulink-PS Converter2/RConn1 -- Rectangular Joint/LConn3
  PS-Simulink Converter12/LConn1 -- SimScape SimMechanics Interface/LConn1
